simulink model "controller2_SR"  (R2020a)
settings: Solver=VariableStepAuto  StartTime=0.0  StopTime=30.0  RelTol=1e-3
values from neighbouring files (symbols this model uses):
  A = [0,       1 ... (first row only)    [capt_init_model.m]    (also in human_init_model.m; sofia_udp_test.m = [0 1; -k/J -b/J])
  b = 0.05    [sofia_udp_test.m]
  B = [0 ... (first row only)    [capt_init_model.m]    (also in human_init_model.m; sofia_udp_test.m = [0; 1/J])
  C = [1, 0]    [capt_init_model.m]    (also in human_init_model.m; sofia_udp_test.m = [1 0])
  D = 0    [capt_init_model.m]    (also in human_init_model.m; sofia_udp_test.m = zeros())
  k = 13.14    [sofia_udp_test.m]
  omega_c = 62    [sofia_udp_test.m]
  Ts = mean(diff(seg_time))    [capt_est_params.m]    (also in capt_fidelity.m = mean(diff(time_data)); sofia_udp_test.m = 0.001)
undefined symbols (not defined in the file or in its folder): den_d, DiscIntNeverNeededParam, num_d
libraries: etargetslib x1, instrumentlib x1
settings Model: Creator=javot  LastModifiedBy=javot

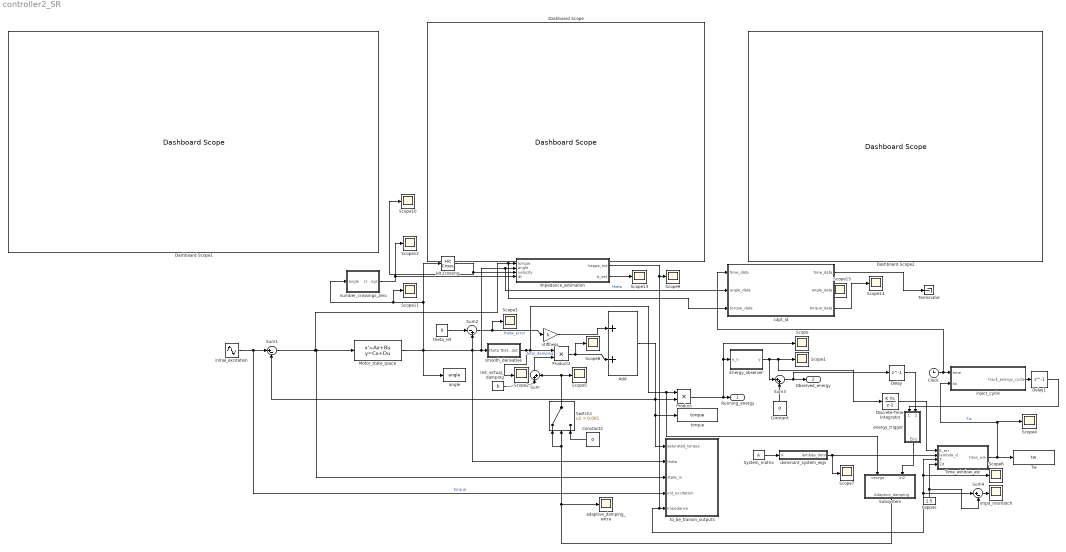
== system controller2_SR ==
  Add : Sum
  Clock : Clock
  Constant : Constant  Value=0
  Constant2 : Constant  Value=0
  Dashboard Scope : DashboardScope
  Dashboard Scope1 : DashboardScope
  Dashboard Scope2 : DashboardScope
  Delay : Delay  DelayLength=1
  Delay1 : Delay  DelayLength=1
  Discrete-Time Integrator : DiscreteIntegrator  gainval=deltaT  SampleTime=-1  ICPrevOutput=DiscIntNeverNeededParam  ICPrevScaledInput=DiscIntNeverNeededParam
  Energy_observer : MATLAB Function  TreatAsAtomicUnit=on
  Hit Crossing : HitCross
  Init_virtual_damping : Constant  Value=b
  Motor_state_space : StateSpace  A=A  B=B  C=C  D=D  InitialCondition=0  ContinuousStateAttributes="\"\""
  Product : Product
  Product2 : Product
  Scope{,1..15} (16 alike) : Scope
  Subsystem : Subsystem
  Sum : Sum  Inputs=|++
  Sum1 : Sum  Inputs=|+-
  Sum2 : Sum  Inputs=|-+
  Sum3 : Sum  Inputs=|++
  Sum4 : Sum  Inputs=|+-
  Switch1 : Switch  Criteria=u2 > Threshold  Threshold=0.001
  System_matrix : Constant  Value=A
  Terminator : Terminator
  Time_window_est : MATLAB Function  TreatAsAtomicUnit=on
  Tw : ToWorkspace  VariableName=tw  SaveFormat=Timeseries  SampleTime=-1
  adaptive_damping_extra : Scope
  angle : ToWorkspace  VariableName=angle  SaveFormat=Timeseries  SampleTime=-1
  capt_id : MATLAB Function  TreatAsAtomicUnit=on
  dominant_system_eigs : MATLAB Function  TreatAsAtomicUnit=on
  energy_trigger : MATLAB Function  TreatAsAtomicUnit=on
  impd_mismatch : Scope
  impedance_estimation : MATLAB Function  TreatAsAtomicUnit=on
  initial_excitation : Sin  SampleTime=Ts
  inject_cycle : MATLAB Function  TreatAsAtomicUnit=on
  kappas : Constant  Value=1.5
  number_crossings_zero : MATLAB Function  TreatAsAtomicUnit=on
  smooth_derivative : Subsystem
  stiffness : Gain  Gain=k
  theta_ref : Constant  Value=0
  to_be_transm_outputs : Subsystem
  torque : ToWorkspace  VariableName=torque  SaveFormat=Timeseries  SampleTime=-1
  Running_energy : Outport
  Observed_energy : Outport  Port=2
  wires:
  Sum2/1 -> Scope3/1, stiffness/1  "theta_error"
  Sum1/1 -> to_be_transm_outputs/3(state_in), Motor_state_space/1, capt_id/3("torque_data "), impedance_estimation/1(torque)
  Energy_observer/1(y) -> Sum3/1, Discrete-Time Integrator/1, Scope1/1
  stiffness/1 -> Add/1
  Sum3/1 -> Delay/1, Observed_energy/1
  initial_excitation/1 -> to_be_transm_outputs/4(init_excitation), Sum1/1  "torque"
  Constant/1 -> Sum3/2
  Product/1 -> Scope/1, Energy_observer/1(e_n), Running_energy/1
  Motor_state_space/1 -> capt_id/2("angle_data "), impedance_estimation/2(angle), smooth_derivative/1(theta), to_be_transm_outputs/2(theta), Sum2/2, angle/1, Hit Crossing/1, Scope11/1, number_crossings_zero/1(angle)  "theta"
  Add/1 -> Product/2, Sum1/2, torque/1, to_be_transm_outputs/1(saturated_torque)
  Product2/1 -> Scope8/1, Add/2
  theta_ref/1 -> Sum2/1
  Init_virtual_damping/1 -> Sum/1
  Sum/1 -> Product2/2  "total_damping"
  System_matrix/1 -> dominant_system_eigs/1(A)
  dominant_system_eigs/1(lambda_dom) -> Scope7/1, Time_window_est/2(lambda_d)
  Time_window_est/1(time_win) -> Tw/1, inject_cycle/2(tw), Scope4/1  "Tw"
  Switch1/1 -> Sum/2, Scope5/1
  Constant2/1 -> Switch1/3
  smooth_derivative/1(theta_dot) -> Scope2/1, Subsystem/1(omega), Product/1, Product2/1
  Discrete-Time Integrator/1 -> Time_window_est/1(E_err)
  Delay/1 -> energy_trigger/2(energy_in)
  energy_trigger/1(Einj) -> Subsystem/2(In2)
  inject_cycle/1(track_energy_cycle) -> Delay1/1
  Delay1/1 -> energy_trigger/1(trigger)
  Subsystem/1(Adaptive_damping) -> adaptive_damping_extra/1, Switch1/1, Switch1/2
  Sum4/1 -> impd_mismatch/1
  kappas/1 -> Sum4/2, Time_window_est/4(Zd)
  number_crossings_zero/1(crossings) -> Scope12/1, impedance_estimation/4(dt)
  impedance_estimation/1(kappa_est) -> Time_window_est/3(Z), Scope6/1, Sum4/1, to_be_transm_outputs/5(impedance), Scope9/1
  Hit Crossing/1 -> Scope10/1, impedance_estimation/3(velocity)
  impedance_estimation/2(b_est) -> Scope13/1
  Clock/1 -> capt_id/1("time_data "), inject_cycle/1(time)
  capt_id/3(torque_data) -> Scope14/1
  capt_id/1(time_data) -> Terminator/1

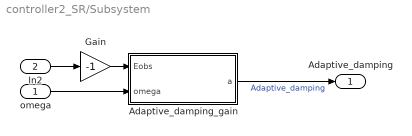
== system controller2_SR/Subsystem ==
  omega : Inport
  In2 : Inport  Port=2
  Adaptive_damping_gain : MATLAB Function  TreatAsAtomicUnit=on
  Gain : Gain  Gain=-1
  Adaptive_damping : Outport
  wires:
  In2/1 -> Gain/1
  Gain/1 -> Adaptive_damping_gain/1(Eobs)
  Adaptive_damping_gain/1(a) -> Adaptive_damping/1  "Adaptive_damping"
  omega/1 -> Adaptive_damping_gain/2(omega)

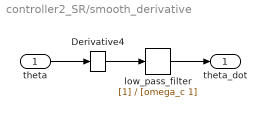
== system controller2_SR/smooth_derivative ==
  theta : Inport
  Derivative4 : Derivative
  low_pass_filter : TransferFcn  Denominator=[omega_c 1]
  theta_dot : Outport
  wires:
  Derivative4/1 -> low_pass_filter/1
  theta/1 -> Derivative4/1
  low_pass_filter/1 -> theta_dot/1

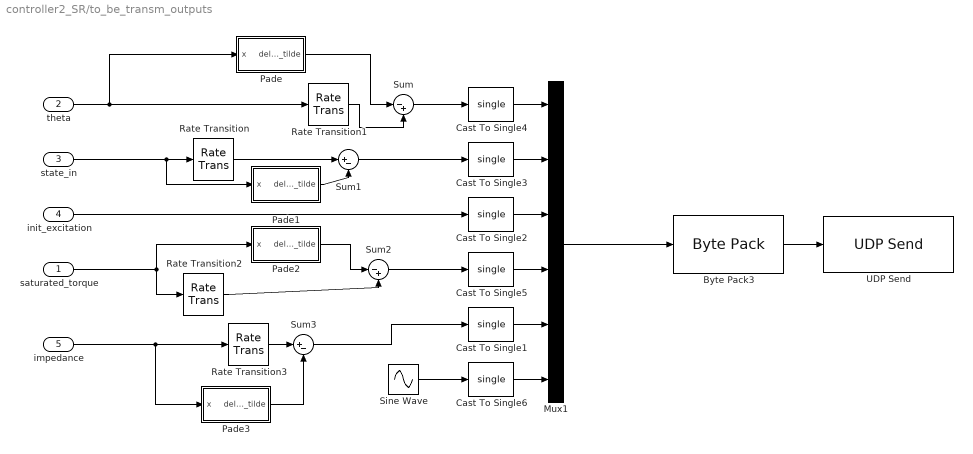
== system controller2_SR/to_be_transm_outputs ==
  saturated_torque : Inport
  theta : Inport  Port=2
  state_in : Inport  Port=3
  init_excitation : Inport  Port=4
  impedance : Inport  Port=5
  Byte Pack3 : etargetslib/Byte Pack  datatypes={'single'}  byteAlign=1
  Cast To Single{1..6} (6 alike) : DataTypeConversion  OutDataTypeStr=single
  Mux1 : Mux  Inputs=6
  Pade : Subsystem
  Pade1 : Subsystem
  Pade2 : Subsystem
  Pade3 : Subsystem
  Rate Transition{,1..3} (4 alike) : RateTransition
  Sine Wave : Sin  SampleTime=0.001
  Sum : Sum  Inputs=|-+
  Sum1 : Sum  Inputs=|+-
  Sum2 : Sum  Inputs=|-+
  Sum3 : Sum  Inputs=|+-
  UDP Send : instrumentlib/UDP Send  Host=134.105.60.99  Port=55001  LocalPort=-1  EnablePortSharing=off  ByteOrder=BigEndian  OutputDatagramPacketSize=512  EnableBlockingMode=on  LocalAddress=0.0.0.0
  wires:
  Byte Pack3/1 -> UDP Send/1
  Mux1/1 -> Byte Pack3/1
  Sine Wave/1 -> Cast To Single6/1
  init_excitation/1 -> Cast To Single2/1
  theta/1 -> Pade/1(x), Rate Transition1/1
  saturated_torque/1 -> Pade2/1(x), Rate Transition2/1
  impedance/1 -> Pade3/1(x), Rate Transition3/1
  Cast To Single4/1 -> Mux1/1
  Cast To Single3/1 -> Mux1/2
  Cast To Single5/1 -> Mux1/4
  Cast To Single2/1 -> Mux1/3
  Cast To Single1/1 -> Mux1/5
  Cast To Single6/1 -> Mux1/6
  Rate Transition1/1 -> Sum/2
  Sum/1 -> Cast To Single4/1
  Rate Transition/1 -> Sum1/1
  Sum1/1 -> Cast To Single3/1
  Rate Transition2/1 -> Sum2/2
  Sum2/1 -> Cast To Single5/1
  Rate Transition3/1 -> Sum3/1
  Sum3/1 -> Cast To Single1/1
  state_in/1 -> Pade1/1(x), Rate Transition/1
  Pade2/1(delay_tilde) -> Sum2/1
  Pade/1(delay_tilde) -> Sum/1
  Pade1/1(delay_tilde) -> Sum1/2
  Pade3/1(delay_tilde) -> Sum3/2

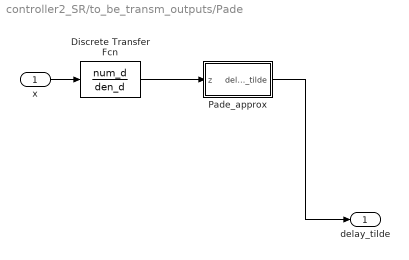
== system controller2_SR/to_be_transm_outputs/Pade ==
  x : Inport
  Discrete Transfer Fcn : DiscreteTransferFcn  Numerator=num_d  Denominator=den_d
  Pade_approx : MATLAB Function  TreatAsAtomicUnit=on
  delay_tilde : Outport
  wires:
  Discrete Transfer Fcn/1 -> Pade_approx/1(z)
  Pade_approx/1(delay_tilde) -> delay_tilde/1
  x/1 -> Discrete Transfer Fcn/1

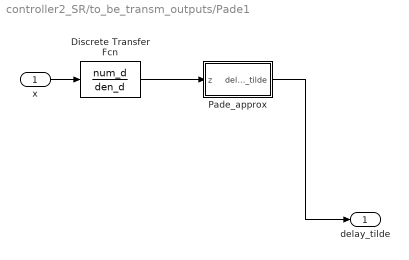
== system controller2_SR/to_be_transm_outputs/Pade1 ==
  x : Inport
  Discrete Transfer Fcn : DiscreteTransferFcn  Numerator=num_d  Denominator=den_d
  Pade_approx : MATLAB Function  TreatAsAtomicUnit=on
  delay_tilde : Outport
  wires:
  Discrete Transfer Fcn/1 -> Pade_approx/1(z)
  Pade_approx/1(delay_tilde) -> delay_tilde/1
  x/1 -> Discrete Transfer Fcn/1

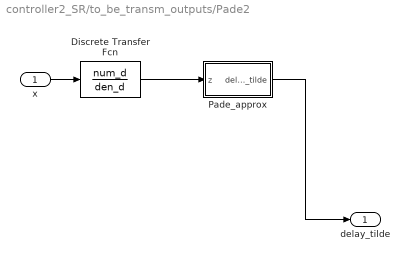
== system controller2_SR/to_be_transm_outputs/Pade2 ==
  x : Inport
  Discrete Transfer Fcn : DiscreteTransferFcn  Numerator=num_d  Denominator=den_d
  Pade_approx : MATLAB Function  TreatAsAtomicUnit=on
  delay_tilde : Outport
  wires:
  Discrete Transfer Fcn/1 -> Pade_approx/1(z)
  Pade_approx/1(delay_tilde) -> delay_tilde/1
  x/1 -> Discrete Transfer Fcn/1

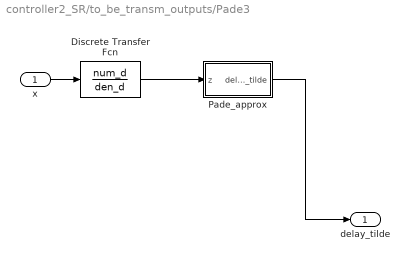
== system controller2_SR/to_be_transm_outputs/Pade3 ==
  x : Inport
  Discrete Transfer Fcn : DiscreteTransferFcn  Numerator=num_d  Denominator=den_d
  Pade_approx : MATLAB Function  TreatAsAtomicUnit=on
  delay_tilde : Outport
  wires:
  Discrete Transfer Fcn/1 -> Pade_approx/1(z)
  Pade_approx/1(delay_tilde) -> delay_tilde/1
  x/1 -> Discrete Transfer Fcn/1

== matlab function controller2_SR/number_crossings_zero ==
  settings: updateMethod=DISCRETE
  data: angle input; crossings output
function crossings = fcn(angle)

persistent prev_angle crossings_count

if isempty(prev_angle)
    prev_angle = angle;
    crossings_count = 0;
end

% Detect sign change (zero crossing)
if (angle > 0 && prev_angle < 0) || (angle < 0 && prev_angle > 0)
    crossings_count = crossings_count + 1;
end

% Update previous value
prev_angle = angle;

% Output
crossings = crossings_count;

end

== matlab function controller2_SR/capt_id ==
  data: time_data output; angle_data output; torque_data output; time_data input; angle_data input; torque_data input
function [time_data, angle_data, torque_data] = capt_id(time_data, angle_data, torque_data)

    % =============================================================
    % 1. PURE STIFFNESS (k-only) THEORETICAL TRANSFER FUNCTION & BODE
    % =============================================================
    J_val = 0.0103;          % Fixed motor inertia
    k_avg = 42.95 + 1;       % Average estimated stiffness
    b_avg = 9.1079;

    num = [1];
    den = [J_val, b_avg, k_avg]; 
    sys_k_only = tf(num, den);

    disp('--- PURE STIFFNESS TRANSFER FUNCTION ---');
    disp(sys_k_only);

    % Plot Theoretical Bode Diagram
    figure('Name', 'k-Only System Bode Diagram');
    bode(sys_k_only);
    grid on;
    title(sprintf('Theoretical Bode Plot (k = %.2f, b = %.2f)', k_avg, b_avg));

    % Ensure input data vectors are column vectors to avoid dimension mismatches
    time_data = time_data(:);
    angle_data = angle_data(:);
    torque_data = torque_data(:);

    % =============================================================
    % 2. EMPIRICAL MODEL & BODE PLOT (Post-processing Recorded Data)
    % =============================================================
    if length(time_data) > 10
        % Calculate uniform sample time
        Ts = mean(diff(time_data));
        
        % Create an iddata object (Input: Torque, Output: Angle)
        data = iddata(angle_data, torque_data, Ts);
        
        % Estimate transfer function model from recorded stream (Empirical)
        % Using 2 poles and 1 zero matching your physical second-order structure
        sys_empirical = tfest(data, 2, 1);
        
        % Generate the Empirical Bode Plot in a new figure window
        figure('Name', 'System Identification - Empirical Bode Plot', 'Position', [200, 200, 700, 500]);
        bode(sys_empirical);
        grid on;
        title('Bode Plot of Empirical dSPACE System');
        disp('Empirical Bode plot generated successfully.');
        
        % =============================================================
        % ACTUAL (THEORETICAL MODEL BASED ON MEASURED DATA) BODE PLOT
        % =============================================================
        sys_actual = tf([1], [J_val, b_avg, k_avg]);
        
        % Generate the Actual/Theoretical Bode Plot in a separate figure window
        figure('Name', 'System Identification - Actual Theoretical Bode Plot', 'Position', [300, 200, 700, 500]);
        bode(sys_actual);
        grid on;
        title(sprintf('Bode Plot of Actual Model (J=%.4f, b=%.4f, k=%.2f)', J_val, b_avg, k_avg));
        disp('Actual theoretical Bode plot generated successfully.');
    else
        disp('Not enough data collected to generate reliable Bode plots.');
    end

    % =============================================================
    % 3. DIRECT NON-PARAMETRIC BODE PLOT (Angle & Torque Measurements Only)
    % =============================================================
    if length(time_data) > 20
        % Calculate uniform sample time and frequency
        dt = mean(diff(time_data));
        Fs = 1 / dt; 
        
        % Detrend data to remove any DC biases or offsets
        torque_clean = detrend(torque_data);
        angle_clean = detrend(angle_data);
        
        % Compute direct Frequency Response Estimate (FRF) using Welch's method.
        % Pass empty brackets [] for default window/noverlap/nfft, followed by Fs.
        [H, freq_vector] = tfestimate(torque_clean, angle_clean, [], [], [], Fs);
        
        % Convert frequency vector from Hz to rad/s for standard Bode plotting
        omega = freq_vector * 2 * pi;
        
        % Convert magnitude to decibels (dB) and phase to degrees
        mag_dB = 20 * log10(abs(H));
        phase_deg = unwrap(angle(H)) * (180 / pi);
        
        % Plot the Direct Measured Bode Diagram
        figure('Name', 'Direct Measured Bode Plot (Angle vs Torque)', 'Position', [200, 200, 700, 600]);
        
        subplot(2,1,1);
        semilogx(omega, mag_dB, 'b-', 'LineWidth', 1.5);
        grid on;
        grid minor;
        ylabel('Magnitude (dB)');
        title('Direct Empirical Bode Plot from Measured Angle & Torque');
        
        subplot(2,1,2);
        semilogx(omega, phase_deg, 'r-', 'LineWidth', 1.5);
        grid on;
        grid minor;
        xlabel('Frequency (rad/s)');
        ylabel('Phase (deg)');
        
        disp('Direct non-parametric Bode plot generated successfully from raw measurements.');
    else
        disp('Not enough data collected to generate a reliable direct Bode plot.');
    end
end

== matlab function controller2_SR/to_be_transm_outputs/Pade1/Pade_approx ==
  data: delay_tilde output; z input
function delay_tilde= fcn(z)
persistent z_prev; 
persistent delay_prev;

if isempty(z_prev)
    z_prev = 0;
    delay_prev = 0;
end
delay_tilde = z/3 + z_prev + (1/3)*delay_prev;
z_prev = z;
delay_prev = delay_tilde;

end

== matlab function controller2_SR/to_be_transm_outputs/Pade/Pade_approx ==
  data: delay_tilde output; z input
function delay_tilde= fcn(z)
persistent z_prev; 
persistent delay_prev;

if isempty(z_prev)
    z_prev = 0;
    delay_prev = 0;
end
delay_tilde = z/3 + z_prev + (1/3)*delay_prev;
z_prev = z;
delay_prev = delay_tilde;

end

== matlab function controller2_SR/to_be_transm_outputs/Pade2/Pade_approx ==
  data: delay_tilde output; z input
function delay_tilde= fcn(z)
persistent z_prev; 
persistent delay_prev;

if isempty(z_prev)
    z_prev = 0;
    delay_prev = 0;
end
delay_tilde = z/3 + z_prev + (1/3)*delay_prev;
z_prev = z;
delay_prev = delay_tilde;

end

== matlab function controller2_SR/to_be_transm_outputs/Pade3/Pade_approx ==
  data: delay_tilde output; z input
function delay_tilde= fcn(z)
persistent z_prev; 
persistent delay_prev;

if isempty(z_prev)
    z_prev = 0;
    delay_prev = 0;
end
delay_tilde = z/3 + z_prev + (1/3)*delay_prev;
z_prev = z;
delay_prev = delay_tilde;

end

== matlab function controller2_SR/Energy_observer ==
  settings: updateMethod=DISCRETE
  data: e_n input; y output
function y = fcn(e_n)

persistent e_prev

if isempty(e_prev)
    e_prev = 0.01;      % initial condition
end

y = e_n - e_prev;

e_prev = y;

== matlab function controller2_SR/inject_cycle ==
  settings: updateMethod=DISCRETE
  data: time input; track_energy_cycle output; tw input
function track_energy_cycle  = fcn(time, tw)

%Induction on time window 
persistent start_time 

if isempty(start_time)
    start_time = 0.0;
end 
if time-start_time>tw 
    track_energy_cycle = true;
    start_time = time;
else
    track_energy_cycle = false;
end 

end

== matlab function controller2_SR/Subsystem/Adaptive_damping_gain ==
  settings: updateMethod=DISCRETE
  data: Eobs input; a output; omega input
function a = fcn(Eobs, omega)

persistent a_prev

%% Parameters
gamma = 0.05;          % adaptation gain (tune 0.01-0.2)
omega_min = 1e-3;      % avoid division by zero

a_min = 0.05;          % minimum damping
a_max = 5.0;           % maximum damping

%% Initialization
if isempty(a_prev)
    a_prev = a_min;
end

%% Safe velocity
omega_safe = max(abs(omega), omega_min);

%% Adaptation

if Eobs < 0

    % Increase damping when passivity is violated
    da = -gamma * Eobs / (omega_safe^2);

    a = a_prev + da;

else

    % Slowly relax damping toward minimum
    relaxation = 0.01;

    a = a_prev - relaxation*(a_prev-a_min);

end

%% Saturation
a = min(max(a,a_min),a_max);

%% Save state
a_prev = a;

end

== matlab function controller2_SR/Time_window_est ==
  settings: updateMethod=DISCRETE
  data: E_err input; time_win output; lambda_d input; Z input; Zd input
function time_win = Time_window_est(E_err, lambda_d, Z, Zd)
%#codegen
% TIME_WINDOW_EST Adaptive observation window estimator using 5-sample time-window
% local minimum detection based on Dinc et al. (IEEE TOH 2024).
%
% Inputs:
%   E_err    : Accumulated energy error/net energy [J]
%   lambda_d : Desired system eigenvalue / dynamic pole
%   Z        : Current impedance estimate
%   Zd       : Target/desired impedance
%
% Output:
%   time_win : Adaptive time window duration [s]

persistent E_window      % 5-sample window: [E(t-2), E(t-1), E(t), E(t+1), E(t+2)]
persistent t_prev        % Previous smoothed window output

%% Limits & Reference Gains
Tmin = 0.01;            % Minimum window time [s]
Tmax = 0.50;            % Maximum window time [s]

tau_min = Tmin;
tau_max = Tmax;

Eref = 1e-3;
k_energy = 0.8;
k_impedance = 0.8;
alpha_time = 0.25;      % Smoothing filter factor

%% Initialization
if isempty(E_window)
    E_window = zeros(5, 1);
    t_prev   = 0.1;
end

%% 1. Slide 5-Sample Time-Window (Fig. 4)
% Shift energy history left: t-2 <- t-1 <- t <- t+1 <- t+2
E_window(1) = E_window(2);
E_window(2) = E_window(3);
E_window(3) = E_window(4);
E_window(4) = E_window(5);
E_window(5) = E_err;

%% 2. Time-Window Local Minimum Detection (Eq. 10)
% Condition: E(t-2) > E(t-1) > E(t) < E(t+1) < E(t+2)
% Validates true energy cycle transition without noise-induced false triggers
is_cycle_min = (E_window(1) > E_window(2)) && ...
               (E_window(2) > E_window(3)) && ...
               (E_window(3) < E_window(4)) && ...
               (E_window(4) < E_window(5));

%% 3. System Time Constant Calculation
lambda_real = real(lambda_d);

if lambda_real < -1e-6
    tau_c = -1/lambda_real;
else
    tau_c = tau_max;
end

tau_c = min(max(tau_c, tau_min), tau_max);

%% 4. Normalized Error & Impedance Mismatch
energy_error = abs(E_err) / max(Eref, 1e-12);
impedance_error = norm(Z - Zd) / (norm(Zd) + 1e-12);

% Saturation bounds
energy_error = min(energy_error, 5.0);
impedance_error = min(impedance_error, 5.0);

%% 5. Adaptive Window Scaling (Integrating Paper's Cycle Detection)
% Basic error factor based on energy and impedance mismatch
error_factor = 1.0 / (1.0 + k_energy * energy_error + k_impedance * impedance_error);

% If time-window validates an energy cycle completion (local minimum),
% we confirm dynamic stability and scale toward the nominal target window.
if is_cycle_min
    cycle_factor = 1.0; 
else
    % During transient/noisy phases without cycle minimum, reduce window size
    cycle_factor = 0.5; 
end

% Combine candidate time window
time_candidate = tau_c * error_factor * cycle_factor;
time_candidate = min(max(time_candidate, Tmin), Tmax);

%% 6. Smooth Output Transition
time_win = (1.0 - alpha_time) * t_prev + alpha_time * time_candidate;
time_win = min(max(time_win, Tmin), Tmax);

t_prev = time_win;

end

== matlab function controller2_SR/dominant_system_eigs ==
  data: A input; lambda_dom output
function lambda_dom = fcn(A)

%Fetch eigs of system matrix and find the dominant one 
lambdas = eig(A);
[~, idx]= max(real(lambdas));
lambda_dom = lambdas(idx);

== matlab function controller2_SR/impedance_estimation ==
  settings: updateMethod=DISCRETE
  data: torque input; angle input; velocity input; dt input; kappa_est output; b_est output
function [kappa_est, b_est] = Continuous_Impedance_Estimator(torque, angle, velocity, dt)
%#codegen
% CONTINUOUS RECURSIVE LEAST SQUARES (RLS) IMPEDANCE ESTIMATOR
%
% Dynamically estimates stiffness (kappa) and damping (b) anywhere in the workspace
% without division-by-zero, singular spikes, or zero-crossing distortion.

%% Persistent Estimator States
persistent theta_vec    % Parameter vector [kappa; b]
persistent P            % Estimation covariance matrix (2x2)
persistent lambda_r     % Forgetting factor (0.95 to 0.99)

%% Initialization
if isempty(theta_vec)
    theta_vec = [1.816; 0.01]; % Initial guess for [kappa; b]
    P         = 10.0 * eye(2); % Initial uncertainty matrix
    lambda_r  = 0.98;          % Exponential forgetting factor
end

%% 1. Regressor Matrix (Phi = [angle, velocity])
phi = [angle; velocity];

%% 2. Prediction Error
% Measured torque vs model-predicted torque
torque_pred = phi' * theta_vec;
e_error     = torque - torque_pred;

%% 3. Dynamic Gain & Covariance Update
% Regressor energy check: update ONLY when there is motion/displacement
reg_energy = phi' * phi;

if reg_energy > 1e-8
    % Kalman Gain update: K = P * phi / (lambda + phi' * P * phi)
    den = lambda_r + phi' * P * phi;
    K   = (P * phi) / den;
    
    % Parameter update
    theta_vec = theta_vec + K * e_error;
    
    % Covariance update (P = (I - K*phi')*P / lambda)
    P = (eye(2) - K * phi') * P / lambda_r;
    
    % Enforce Covariance Bounding (prevents estimator covariance blow-up)
    if trace(P) > 500
        P = 10.0 * eye(2);
    end
end

%% 4. Non-Negative Physical Constraints
% Stiffness kappa and damping b must remain non-negative
theta_vec(1) = max(0.0, theta_vec(1)); % kappa >= 0
theta_vec(2) = max(0.0, theta_vec(2)); % b >= 0

%% 5. Output Extraction
kappa_est = theta_vec(1);
b_est     = theta_vec(2);

end

== matlab function controller2_SR/energy_trigger ==
  data: trigger input; Einj output; energy_in input
function Einj = fcn(trigger, energy_in)

if trigger == true
    Einj = energy_in;
else 
    Einj = 0;
end

end
